simulink model "oz_weather"  (R2024a)
settings: Solver=VariableStepAuto  StartTime=0.0  StopTime=10000  RelTol=1e-3
settings Model: Creator=alexandr  LastModifiedBy=alexandr

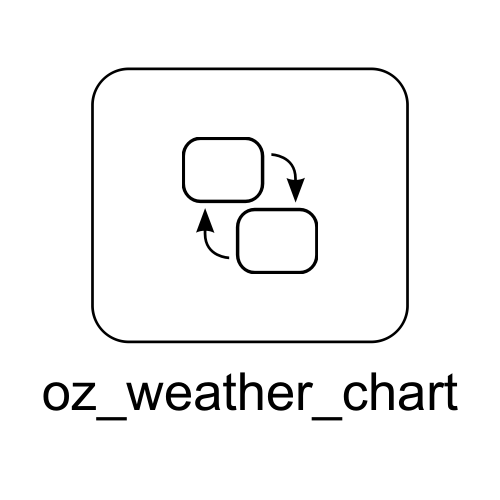
[thumbnail: Simulink's stored preview of the top-level diagram]
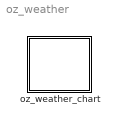
== system oz_weather ==
  oz_weather_chart : Stateflow chart  TreatAsAtomicUnit=on

== stateflow chart oz_weather/oz_weather_chart ==
  state Sunny/
    entry:n_sunny = n_sunny + 1;
  state Rainy/
    entry:n_rainy = n_rainy + 1;
  state Snowy/
    entry:n_snowy = n_snowy + 1;
  (junction 20) -> (junction 22) [order 1] : [(rand(1) > 0.2)]
  (default) -> Sunny : /{n_sunny=0;
      | n_rainy=0;
      | n_snowy=0;}
  (junction 22) -> Sunny [order 1] : [(rand(1) > 0.2)]
  (junction 35) -> Sunny [order 1] : [(rand(1) > 0.5)]
  (junction 22) -> Rainy [order 2]
  Sunny -> (junction 11)
  (junction 33) -> Rainy [order 2]
  (junction 33) -> (junction 35) [order 1] : [(rand(1) > 0.2)]
  (junction 20) -> Snowy [order 2]
  Rainy -> (junction 33)
  (junction 35) -> Snowy [order 2]
  Snowy -> (junction 20)
  (junction 11) -> Rainy [order 2]
  (junction 11) -> Snowy [order 1] : [(rand(1) > 0.5)]
  data: n_rainy local; n_snowy local; n_sunny local
